simulink library "mci_models"  (R2022b)
settings: Solver=VariableStepAuto  StartTime=0.0  StopTime=10.0  RelTol=1e-3
undefined symbols (not defined in the file or in its folder): x0
(part 2 of 2)

== matlab function mci_models/Electric Systems/Magnetic Levitation/MATLAB Function ==
  data: u input; xdot output size=[3,1]; x input; p parameter
function xdot = fcn(u,x,p)

xdot=zeros(size(x));

xdot(1)=x(2);
xdot(2)=p.g-p.L1*x(3)^2/(2*p.m*p.y0*(1+x(1)/p.y0)^2);
xdot(3)=(u-(p.R-p.L1*x(2)/((1+x(1)/p.y0)^2*p.y0))*x(3))/(p.L0+p.L1/(1+x(1)/p.y0));
%xdot(3)=(u-p.R*x(3))/(p.L0+p.L1/(1+x(1)/p.y0));

== matlab function mci_models/Fluid Systems/Pneumatic Cylinder/MATLAB Function ==
  data: u input; dx output; x input; p parameter
function dx = fcn(u,x,p)
%#codegen

dx=zeros(size(x));

dx(1) = x(2);
dx(2) = (p.A*x(3)-p.b*x(2)-p.k*x(1))/p.m;
dx(3) = x(3)/x(1)*(u/p.A-x(2));

== matlab function mci_models/Mechanical Systems/Elevator/MATLAB Function ==
  data: M input; xdot output; x input; p parameter; e output
function [xdot,e] = pendulum_model(M,x,p)

% x=[y;phi;ydot;phidot]

xdot=zeros(size(x));

Fr=p.b1*x(3);
Mr=p.b2*x(4);
l=p.r*x(2);
e=max(0,(x(1)-l)/(l));
Fs=e*p.k;

xdot(1)=x(3);
xdot(2)=x(4);
xdot(3)=p.g-(Fs+Fr)/p.m;
xdot(4)=(Fs*p.r+M-Mr)/p.J;

== matlab function mci_models/Vehicle Systems/Wheel Dynamics/MATLAB Function ==
  data: M input; F input; a output; p parameter
function a = fcn(M,F,p)

a=(M-F*p.r)/p.J;

== matlab function mci_models/Auxiliary Functions/Friction model/MATLAB Function ==
  data: l output; v input; m output; w input; p parameter
function [l,m] = fcn(v,w,p)

% slip
l=(w-v)/v;

% friction model
m=sign(l)*(p.c(1)*(1-exp(-p.c(2)*abs(l)))-p.c(3)*abs(l))*exp(-p.c(4)*abs(v));

== matlab function mci_models/Pendula/Motion Controlled Pendulum/MATLAB Function ==
  data: v input; a input; xdot output; x input; p parameter
function xdot = pendulum_model(v,a,x,p)

% x=[x;phi;phidot]

xdot=zeros(size(x));

xdot(1)=v;
xdot(2)=x(3);
xdot(3)=-p.m1*p.s*(sin(x(2))*p.g+cos(x(2))*a)/(p.J1+p.m1*p.s^2)

== matlab function mci_models/Auxiliary Functions/Trajectory/tragen ==
  data: y output; t input; p parameter; dy output; ddy output
function [y,dy,ddy] = fcn(t,p)

if t<p.t1
    y=p.y1;
    dy=0;
    ddy=0;
elseif t>p.t2
    y=p.y2;
    dy=0;
    ddy=0;
else
    y=p.y1+(p.y2-p.y1)*polyval(p.p,(t-p.t1)/p.dt);
    dy=(p.y2-p.y1)*polyval(p.dp,(t-p.t1)/p.dt)/p.dt;
    ddy=(p.y2-p.y1)*polyval(p.ddp,(t-p.t1)/p.dt)/p.dt^2;
end

== matlab function mci_models/Fluid Systems/Fan Model/Sensor1/Triggered Subsystem/MATLAB Function ==
  data: phi input; w output; T parameter
function w = fcn(phi,T)

persistent phi_o

if isempty(phi_o)
    phi_o=0;
end

w = (phi-phi_o)/T;
phi_o=phi;

== matlab function mci_models/Fluid Systems/Fan Model/Sensor2/Triggered Subsystem/MATLAB Function ==
  data: phi input; w output; T parameter
function w = fcn(phi,T)

persistent phi_o

if isempty(phi_o)
    phi_o=0;
end

w = (phi-phi_o)/T;
phi_o=phi;

== matlab function mci_models/Pendula/Pendulum on Cart/MATLAB Function ==
  data: F input; xdot output; x input; p parameter
function xdot = pendulum_model(F,x,p)

% x=[x;xdot;phi;phidot]

xdot=zeros(size(x));

Fr=p.b0*x(3);

xdot(1)=x(3);
xdot(2)=x(4);
xdot(3)=((p.m1*p.s^2+p.J)*(F-Fr+p.m1*p.s*sin(x(2))*x(4)^2)+...
    (p.m1*p.g*p.s*sin(x(2))+x(4)^2*p.b1)*p.m1*p.s*cos(x(2)))/...
    ((p.m0+p.m1)*(p.m1*p.s^2+p.J)-(p.m1*p.s*cos(x(2)))^2);
xdot(4)=(-(p.m0+p.m1)*(p.m1*p.g*p.s*sin(x(2))+x(4)*p.b1)-...
    (F-Fr+p.m1*p.s*x(4)^2*sin(x(2)))*p.m1*p.s*cos(x(2)))/...
    ((p.m0+p.m1)*(p.m1*p.s^2+p.J)-(p.m1*p.s*cos(x(2)))^2);

== matlab function mci_models/Pendula/Mathematical Pendulum/MATLAB Function ==
  data: u input; xdot output; x input; p parameter
function xdot = fcn(u,x,p)

xdot=zeros(size(x));

xdot(1)=x(2);
xdot(2)=(u-p.k*x(1)-p.b*x(2)-p.g*p.m*p.l*sin(x(1)))/(p.m*p.l^2);

== matlab function mci_models/DC-DC Converters/Cuk Converter/Cuk converter1 ==
  data: d input; dx output; x input; p parameter
function dx = fcn(d,x,p)
%#codegen

A=[-p.R1/p.L1 0 -(1-d)/p.L1 0; ...
    0 -p.R2/p.L2 -d/p.L2 -1/p.L2; ...
    (1-d)/p.C1 d/p.C1 0 0; ...
    0 1/p.C2 0 -p.G/p.C2];
B=[1/p.L1;0;0;0];

dx=zeros(4,1);
dx=A*x+B*p.ui;

== matlab function mci_models/Vehicle Systems/Car Dynamics/MATLAB Function ==
  data: F input; a output; phi input; v input; p parameter
function a = fcn(F,phi,v,p)

a=(F-p.cd*p.rho*v^2*p.A/2)/p.m-p.g*(p.cf+sin(phi));

== matlab function mci_models/Auxiliary Functions/Polynomial/MATLAB Function1 ==
  data: y output; u input; p parameter
function y = fcn(u,p)

y=polyval(p,u);

== matlab function mci_models/Vehicle Systems/Car Kinematics/MATLAB Function ==
  data: v input; xdot output; phi input; x input; l parameter
function xdot = fcn(v,phi,x,l)

xdot=zeros(size(x));

xdot(1)=v*cos(x(3));
xdot(2)=v*sin(x(3));
xdot(3)=v*tan(phi)/l;

== matlab function mci_models/Fluid Systems/Tank with Outflow/MATLAB Function ==
  data: qo output; qi input; hdot output; h input; p parameter
function [qo,hdot] = fcn(qi,h,p)

qo=sqrt(2*p.g*h/(1+p.zeta))*p.Ao*p.rho;
hdot = (qi-qo)/(p.rho*p.At);

== matlab function mci_models/Mechanical Systems/Segway Model/MATLAB Function ==
  data: u input; x input; dx output; p parameter
function dx = fcn(u,x,p)

dx=zeros(4,1);


dx(1) = x(3);   % alpha
dx(2) = x(4);   % theta
dx(3) = ((p.I1-p.I01*cos(x(2)))*u+p.I1*p.I01*sin(x(2))*x(4)^2-(p.I1-p.I01*cos(x(2)))*p.b1*x(4)-((1+p.nu)*p.I1-p.I01*cos(x(2)))*p.b1*x(3)+p.I01^2*p.g*sin(x(2))*cos(x(2)))/(p.I0*p.I1-p.I01^2*cos(x(2))^2);     % d(alpha)
dx(4) = ((p.I0-p.I01*cos(x(2)))*u-p.I01^2*sin(x(2))*cos(x(2))*x(4)^2-(p.I0-p.I01*cos(x(2)))*p.b1*x(4)-(p.I0-p.I01*(1+p.nu)*cos(x(2)))*p.b1*x(3)-p.I0*p.I01*p.g*sin(x(2)))/(p.I0*p.I1-p.I01^2*cos(x(2))^2);     % d(theta)

== matlab function mci_models/Mechanical Systems/Lunar Lander/MATLAB Function ==
  data: u input; xdot output; x input; p parameter
function xdot = fcn(u,x,p)

xdot=zeros(size(x));

xdot(1)=x(2);
xdot(2)=-p.g+p.vt/x(3)*u;
xdot(3)=-u;
